simulink subsystem "block_control"  (R2019b)
settings: Solver=VariableStepAuto  StartTime=0.0  StopTime=10.0  RelTol=1e-3
libraries: blocklib x1
settings Model: Creator=imanol  LastModifiedBy=imanol

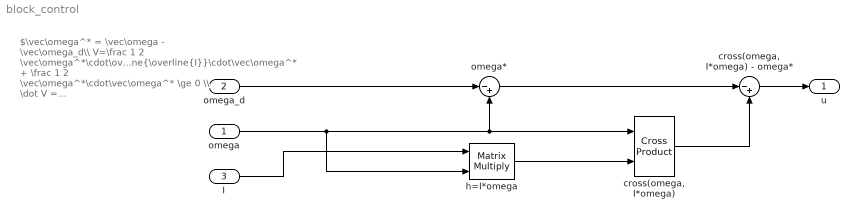
== system block_control ==
  note: $\vec\omega^* = \vec\omega - \vec\omega_d\\ V=\frac 1 2 \vec\omega^*\cdot\overline{\overline{I}}\cdot\vec\omega^* + \frac 1 2 \vec\omega^*\cdot\vec\omega^* \ge 0 \\ \dot V = \dot{\vec\omega}\cdot\left[\overline{\overline{I}}\cdot\vec\omega^* + \vec\omega^*\right] =\\ \overline{\overline{I}}^{-1}\left[\vec u - \vec\omega\times\overline{\overline{I}}\cdot\vec\omega\right]\left[\overline{\overline{I}}\cdot\vec\omega^* + \vec\omega^*\right] \\ \vec u = \vec\omega\times\overline{\overline{I}}\cdot\vec\omega-\vec\omega^*\\ \dot V = \overline{\overline{I}}^{-1}\left[-\vec\omega^*\right]\left[\overline{\overline{I}}\cdot\vec\omega^* + \vec\omega^*\right] \\ \dot V = -\overline{\overline{I}}^{-1} \left[ \vec\omega^* \cdot \overline{\overline{I}}\cdot\vec\omega^* + \vec\omega^*\cdot\vec\omega^* \right] \le 0$
  omega : Inport  Unit=rad/sec  PortDimensions=[3,1]
  omega_d : Inport  Port=2  Unit=rad/sec  PortDimensions=[3,1]
  I : Inport  Port=3  Unit=kg*m*m*m*m  PortDimensions=[3,3]
  "cross(omega, I*omega)" : blocklib/Cross Product  SystemSampleTime=-1  Latency=0  AutoFrameSizeCalculation=off
      settings: SourceProductName=Custom Library
  "cross(omega, I*omega) - omega*" : Sum  Inputs=|-+
  h=I*omega : Product  Multiplication=Matrix(*)
  omega* : Sum  Inputs=|-+
  u : Outport  VectorParamsAs1DForOutWhenUnconnected=off
  wires:
  omega_d/1 -> omega*/1
  I/1 -> h=I*omega/1
  "cross(omega, I*omega)"/1 -> "cross(omega, I*omega) - omega*"/2
  omega/1 -> h=I*omega/2, omega*/2, "cross(omega, I*omega)"/1
  h=I*omega/1 -> "cross(omega, I*omega)"/2
  omega*/1 -> "cross(omega, I*omega) - omega*"/1
  "cross(omega, I*omega) - omega*"/1 -> u/1
